simulink model "Stepper_Serial"  (R2021a)
settings: Solver=VariableStepAuto  StartTime=0.0  StopTime=Inf  RelTol=1e-3  EnableMultiTasking=on
undefined symbols (not defined in the file): LF
libraries: instrumentseriallib x3, etargetslib x1
settings Model: SILPILModeSetting=veronly  ExtModeTrigDuration=2  Creator=Waseem Sajjad  LastModifiedBy=Waseem Sajjad
settings RTWCC: BuildConfiguration=Faster Runs

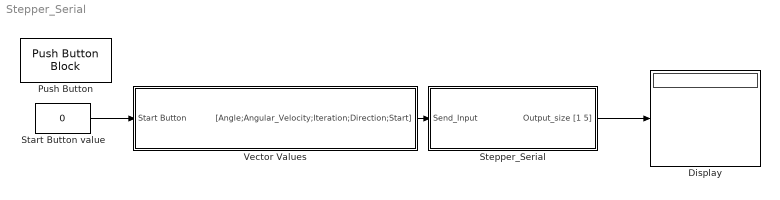
== system Stepper_Serial ==
  Display : Display
  Push Button : PushButtonBlock  LabelPosition=Top
  Start Button value : Constant  Value=0
  Stepper_Serial : Subsystem
  Vector Values : Subsystem  mask{P=300, S=300.0, I=5, D=Anticlockwise}
      mask prompts: P "Angle (deg)"; S "Angular Velocity (RPM)"; I "Iteration"; D "Direction"
      mask TypeOptions D: Anticlockwise | Clockwise
  wires:
  Vector Values/1("[Angle;Angular_Velocity;Iteration;Direction;Start]") -> Stepper_Serial/1(Send_Input)
  Stepper_Serial/1(Output_size [1 5]) -> Display/1
  Start Button value/1 -> Vector Values/1(Start Button)

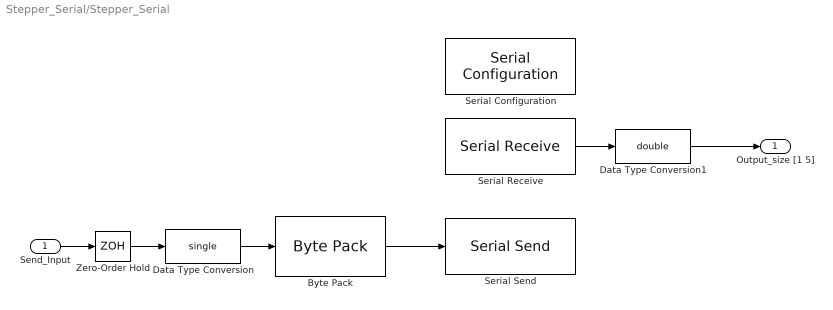
== system Stepper_Serial/Stepper_Serial ==
  Send_Input : Inport
  Byte Pack : etargetslib/Byte Pack  datatypes={'single'}  byteAlign=4
  Data Type Conversion : DataTypeConversion  OutDataTypeStr=single
  Data Type Conversion1 : DataTypeConversion  OutDataTypeStr=double
  Serial Configuration : instrumentseriallib/Serial Configuration  Priority=-200000  Port=COM3  ComPort=COM3  BaudRate=115200  DataBits=8  Parity=none  StopBits=1  ByteOrder=little-endian  FlowControl=none  Timeout=1  SimulateUsing=Interpreted execution  BlockInModel=on
  Serial Receive : instrumentseriallib/Serial Receive  Priority=1  Port=COM3  ComPort=COM3  DataType=single  SaveDataType=uint8  ToggleHeader=on  Header='A'  ToggleTerminator=on  Terminator=LF ('\n')  CustomTerminator=[]  ToggleDataSize=on  DataSize=[1 5]  EnableBlockingMode=on  ActionDataUnavailable=Output last received value  ActionWhenDataUnavailable=Output last received value  CustomValue=0  SampleTime=0.05  SimulateUsing=Interpreted execution  BlockInModel=on
  Serial Send : instrumentseriallib/Serial Send  Priority=1  Port=COM3  ComPort=COM3  Header=[]  Terminator=<none>  CustomTerminator=[]  EnableBlockingMode=on  SimulateUsing=Interpreted execution  BlockInModel=on
  Zero-Order Hold : ZeroOrderHold  SampleTime=0.05
  Output_size [1 5] : Outport
  wires:
  Data Type Conversion/1 -> Byte Pack/1
  Zero-Order Hold/1 -> Data Type Conversion/1
  Data Type Conversion1/1 -> Output_size [1 5]/1
  Byte Pack/1 -> Serial Send/1
  Send_Input/1 -> Zero-Order Hold/1
  Serial Receive/1 -> Data Type Conversion1/1

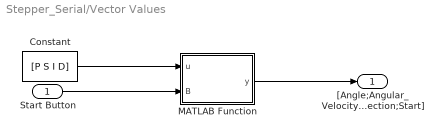
== system Stepper_Serial/Vector Values ==
  Start Button : Inport
  Constant : Constant  Value=[P S I D]
  MATLAB Function : MATLAB Function  TreatAsAtomicUnit=on
  "[Angle;Angular_Velocity;Iteration;Direction;Start]" : Outport
  wires:
  MATLAB Function/1(y) -> "[Angle;Angular_Velocity;Iteration;Direction;Start]"/1
  Constant/1 -> MATLAB Function/1(u)
  Start Button/1 -> MATLAB Function/2(B)

== matlab function Stepper_Serial/Vector Values/MATLAB Function ==
  data: u input; y output; B input
function y = fcn(u, B)
step=u(1)/1.8;
delay=150000/u(2);
y = [step delay u(3) u(4) B];
